simulink model "Full_Model_D_R6"  (R2013a)
settings: Solver=ode45  StartTime=0.0  StopTime=sim_length  MaxStep=1e-4  RelTol=1e-3
values from neighbouring files (symbols this model uses):
  A_Height_d = [1  0.02  0.00306066709295; 0  1  0.292172619905; 0  0  0.751477293075]    [Height_Controller_SS_D_Data.mat]    (also in Height_Controller_Sample_Time.m = A_d)
  A_Roll_d = [1  0.02  0.00957373027909; 0  1  0.913912481482; 0  0  0.751477293075]    [Roll_Controller_SS_D_Data.mat]    (also in Roll_Controller_Sample_Time.m = A_d)
  A_x_d = [1  0.725237004499; 0  0.506103765926]    [xy_Controller_PD_D_Data.mat]    (also in xy_Controller_PID_D_Data.mat; xy_Controller_Sample_Time.m = sys_d.a; xy_Controller_Sample_Time_2.m = sys_d.a)
  A_Yaw_d = [1  0.02  0.000714353321797; 0  1  0.0681924806681; 0  0  0.751477293075]    [Yaw_Controller_SS_D_Data.mat]    (also in Yaw_Controller_Sample_Time.m = A_d)
  B_Height_d = [0.000298297262238 0.0437238156136 0.248522706925]    [Height_Controller_SS_D_Data.mat]    (also in Height_Controller_Sample_Time.m = B_d)
  B_Roll_d = [0.000933070289885 0.136767575416 0.248522706925]    [Roll_Controller_SS_D_Data.mat]    (also in Roll_Controller_Sample_Time.m = B_d)
  B_x_d = [3.95796081795 7.11457501414]    [xy_Controller_PD_D_Data.mat]    (also in xy_Controller_PID_D_Data.mat; xy_Controller_Sample_Time.m = sys_d.b; xy_Controller_Sample_Time_2.m = sys_d.b)
  B_Yaw_d = [7.15569400366e-05 0.0103985455153 0.248522706925]    [Yaw_Controller_SS_D_Data.mat]    (also in Yaw_Controller_Sample_Time.m = B_d)
  C_Height_d = [1 0 0]    [Height_Controller_SS_D_Data.mat]    (also in Height_Controller_Sample_Time.m = C_d)
  C_Roll_d = [1  0  0; 0  1  0]    [Roll_Controller_SS_D_Data.mat]    (also in Roll_Controller_Sample_Time.m = C_d)
  C_x_d = [1 0]    [xy_Controller_PD_D_Data.mat]    (also in xy_Controller_PID_D_Data.mat; xy_Controller_Sample_Time.m = sys_d.c; xy_Controller_Sample_Time_2.m = sys_d.c)
  C_Yaw_d = [1  0  0; 0  1  0]    [Yaw_Controller_SS_D_Data.mat]    (also in Yaw_Controller_Sample_Time.m = C_d)
  coeff_speed1 = [-597.852411164 15567.4958959 -112629.522245 385376.825444 -722286.582234 762343.511164 -424427.181206 96698.0914793]    [Model_Parameters.mat]
  coeff_speed2 = [-33137.8630803 359389.817861 -1655728.0128 4197976.53355 -6322358.45977 5652250.74311 -2774846.33743 576528.840344]    [Model_Parameters.mat]
  coeff_speed3 = [-11936.4686056 137218.314774 -666283.661319 1770733.67902 -2780453.20018 2577948.57948 -1305141.01347 277978.291866]    [Model_Parameters.mat]
  coeff_speed4 = [-6669.45808334 79913.0612752 -401123.444791 1094619.31774 -1754742.75761 1652252.04897 -844945.337957 180729.993964]    [Model_Parameters.mat]
  coeff_thrust1 = [411.996230985 -4101.92524784 17203.3662669 -39329.1303747 52812.747408 -41528.8245566 17635.526271 -3103.13769268]    [Model_Parameters.mat]
  coeff_thrust2 = [3.52133616408 187.041584587 -1860.27738451 7135.94114535 -14212.0789042 15650.5208884 -9059.28758852 2154.75680942]    [Model_Parameters.mat]
  coeff_thrust3 = [-509.084474191 5539.72556164 -25664.1372161 65589.3028623 -99834.0669633 90481.3955019 -45198.9623282 9597.06354792]    [Model_Parameters.mat]
  coeff_thrust4 = [270.975135723 -2599.21496486 10453.4946669 -22770.946547 28872.4244579 -21147.1170047 8185.59308918 -1264.84197054]    [Model_Parameters.mat]
  Drag = 4.45306861536e-07    [Model_Parameters.mat]
  F_Roll_d = A_Roll_d-G_Roll_d*C_Roll_d    [Script_Controller_Sample_Time.m]    (also in Test_Controller_Sample_Time.m)
  F_yIntercept = -10.4432883127    [Model_Parameters.mat]
  Feed_Forward_Height_d = 2    [Height_Controller_SS_D_Data.mat]    (also in Height_Controller_Sample_Time.m)
  Feed_Forward_Roll_d = 0.125    [Roll_Controller_SS_D_Data.mat]    (also in Roll_Controller_Sample_Time.m)
  Feed_Forward_Yaw_d = 0    [Yaw_Controller_SS_D_Data.mat]    (also in Yaw_Controller_Sample_Time.m)
  g = 9.81    [Model_Parameters.mat]
  G_Height_d = [1.56504668046 34.0074022073 8.86962171802]    [Height_Controller_SS_D_Data.mat]    (also in Height_Controller_Sample_Time.m = place(A_d',C_d',P)')
  G_Roll_d = [0.251889913145  0.0200094814614; 0.229685260441  0.24715204306; -0.000711541775691  -9.30790483026e-05]    [Roll_Controller_SS_D_Data.mat]    (also in Roll_Controller_Sample_Time.m = place(A_d',C_d',P)')
  G_x_d = [-0.193896234074 0.15962315642]    [xy_Controller_PD_D_Data.mat]    (also in xy_Controller_PID_D_Data.mat; xy_Controller_Sample_Time.m = place(A_x_d',C_x_d',P)'; xy_Controller_Sample_Time_2.m = place(A_x_d',C_x_d',P)')
  G_Yaw_d = [0.242030648398  0.0200584166088; 0.0044560948779  0.235341919238; -0.000643549416335  -0.000818909263128]    [Yaw_Controller_SS_D_Data.mat]    (also in Yaw_Controller_Sample_Time.m = place(A_d',C_d',P)')
  I_Phi = 0.127422725814    [Model_Parameters.mat]
  I_Psi = 0.236966962973    [Model_Parameters.mat]
  I_Theta = 0.122104044652    [Model_Parameters.mat]
  J = 8e-08    [Model_Parameters.mat]
  K_Height_d = [2.7513802614 0.716922726377 0.637441613793]    [Height_Controller_SS_D_Data.mat]    (also in Height_Controller_Sample_Time.m = K_Height_Reg(1:end-1))
  K_Height_i = -2.03246593773    [Height_Controller_SS_D_Data.mat]    (also in Height_Controller_Sample_Time.m = K_Height_Reg(end))
  K_Roll_d = [2.67637429311 0.450684169535 1.07098831744]    [Roll_Controller_SS_D_Data.mat]    (also in Roll_Controller_Sample_Time.m = K_Roll_Reg(1:end-1))
  K_Roll_i = -2.24117965782    [Roll_Controller_SS_D_Data.mat]    (also in Roll_Controller_Sample_Time.m = K_Roll_Reg(end))
  K_Yaw_d = [1.55130112498 0.960619912039 0.23556072791]    [Yaw_Controller_SS_D_Data.mat]    (also in Yaw_Controller_Sample_Time.m = K_Yaw_Reg(1:end-1))
  K_Yaw_i = -1.12834490639    [Yaw_Controller_SS_D_Data.mat]    (also in Yaw_Controller_Sample_Time.m = K_Yaw_Reg(end))
  Kd_x = 0    [xy_Controller_PD_D_Data.mat]    (also in xy_Controller_PID_D_Data.mat = 0.0186150358972; xy_Controller_Sample_Time.m = get(C,'Kd'); xy_Controller_Sample_Time_2.m = get(C,'Kd'))
  Kd_y = 0    [xy_Controller_PD_D_Data.mat]    (also in xy_Controller_PID_D_Data.mat = 0.0186150358972; xy_Controller_Sample_Time.m = Kd_x; xy_Controller_Sample_Time_2.m = Kd_x)
  Kf = 9.48907430341    [Model_Parameters.mat]
  Ki_x = 0.000229999504243    [xy_Controller_PD_D_Data.mat]    (also in xy_Controller_PID_D_Data.mat = 0.000234605659833; xy_Controller_Sample_Time.m = get(C,'Ki'); xy_Controller_Sample_Time_2.m = get(C,'Ki'))
  Ki_y = 0.000229999504243    [xy_Controller_PD_D_Data.mat]    (also in xy_Controller_PID_D_Data.mat = 0.000234605659833; xy_Controller_Sample_Time.m = Ki_x; xy_Controller_Sample_Time_2.m = Ki_x)
  Kp_x = 0.032529495388    [xy_Controller_PD_D_Data.mat]    (also in xy_Controller_PID_D_Data.mat = 0.0333125747447; xy_Controller_Sample_Time.m = get(C,'Kp'); xy_Controller_Sample_Time_2.m = get(C,'Kp'))
  Kp_y = 0.032529495388    [xy_Controller_PD_D_Data.mat]    (also in xy_Controller_PID_D_Data.mat = 0.0333125747447; xy_Controller_Sample_Time.m = Kp_x; xy_Controller_Sample_Time_2.m = Kp_x)
  Kw = 501.513336009    [Model_Parameters.mat]
  L = 0.338    [Model_Parameters.mat]
  Mass = 2.26    [Model_Parameters.mat]
  Motor_TimeConstant = 0.07    [Model_Parameters.mat]
  NoiseDelay = 0    [All_Controller_Sample_Time.m]
  NoiseMean = 0    [All_Controller_Sample_Time.m]
  omega_0 = (0-F_yIntercept)/Kf    [Test_Controller_Sample_Time.m]    (also in Yaw_Controller_Sample_Time.m = 520)
  omega_Lim = (0-F_yIntercept)/Kf    [Test_Controller_Sample_Time.m]
  Phi_IC = (0/180)*pi    (= 0)    [Test_Controller_Sample_Time.m]
  Pitch_Setpoint = 0    [Test_Controller_Sample_Time.m]
  PropDelay = 0    [All_Controller_Sample_Time.m]
  Psi_IC = (0/180)*pi    (= 0)    [Test_Controller_Sample_Time.m]
  PWM_LimHigher = 2    [Test_Controller_Sample_Time.m]
  PWM_LimLower = 1.1    [Test_Controller_Sample_Time.m]
  Speed_yIntercept = -347.939581678    [Model_Parameters.mat]
  Tau_filter1 = 0.5    [All_Controller_Sample_Time.m]
  Theta_IC = (5/180)*pi    (= 0.0872664625997)    [Test_Controller_Sample_Time.m]
  Ts = 20e-3    (= 0.02)    [All_Controller_Sample_Time.m]
  Ts2 = 1    [All_Controller_Sample_Time.m]
  ViscousDamping = 36*sin(20/180*pi)/8    [All_Controller_Sample_Time.m]
  Yaw_Setpoint = 0    [Test_Controller_Sample_Time.m]
undefined symbols (not defined in the file or in its folder): DiscIntNeverNeededParam
libraries: simulink x9, commnoisgen2 x7
(part 2 of 2)

== system Full_Model_D_R6/Non Linear Quadcopter Model/Motor Model 4 ==
  Duty Cycle : Inport
  1/ Motor Time Constant : Gain  Gain=1/Motor_TimeConstant
  Fcn : Fcn  Expr=coeff_speed4(1)*u(1)^7 + coeff_speed4(2)*u(1)^6+coeff_speed4(3)*u(1)^5 + coeff_speed4(4)*u(1)^4+ coeff_speed4(5)*u(1)^3 +coeff_speed4(6)*u(1)^2+coeff_speed4(7)*u(1)+coeff_speed4(8)
  Fcn1 : Fcn  Expr=coeff_thrust4(1)*u(1)^7 + coeff_thrust4(2)*u(1)^6+coeff_thrust4(3)*u(1)^5 + coeff_thrust4(4)*u(1)^4+ coeff_thrust4(5)*u(1)^3 +coeff_thrust4(6)*u(1)^2+coeff_thrust4(7)*u(1)+coeff_thrust4(8)
  Manual Switch : ManualSwitch
  Manual Switch1 : ManualSwitch  CurrentSetting=0
  Motor 4 : Integrator  InitialCondition=omega_0  LimitOutput=on  LowerSaturationLimit=omega_Lim
  Motor Speed Slope : Gain  Gain=Kw
  Motor Speed Slope1 : Gain  Gain=Kw
  Motor Thrust Slope : Gain  Gain=Kf
  Sum2 : Sum  Inputs=++|
  Sum3 : Sum  Inputs=|+-
  Sum4 : Sum  Inputs=|++
  To Workspace10 : ToWorkspace  VariableName=MotorSpeed1  SampleTime=-1  SaveFormat=Timeseries
  y-Intercept of the  Motor Force Trendline : Constant  Value=F_yIntercept
  y-Intercept of the  Motor Speed Trendline : Constant  Value=Speed_yIntercept
  Thrust : Outport
  Acceleration : Outport  Port=2
  Speed : Outport  Port=3
  wires:
  Motor Thrust Slope/1 -> Sum2/2  "Thrust"
  Motor 4/1 -> Sum3/2, Fcn1/1, Fcn/1, Motor Speed Slope/1, Motor Thrust Slope/1
  Duty Cycle/1 -> Sum3/1
  Sum3/1 -> 1/ Motor Time Constant/1
  1/ Motor Time Constant/1 -> Motor 4/1, Motor Speed Slope1/1
  Motor Speed Slope/1 -> Sum4/1
  Motor Speed Slope1/1 -> Acceleration/1
  Sum2/1 -> Manual Switch1/2
  y-Intercept of the  Motor Force Trendline/1 -> Sum2/1
  Sum4/1 -> Manual Switch/2, To Workspace10/1
  y-Intercept of the  Motor Speed Trendline/1 -> Sum4/2
  Manual Switch/1 -> Speed/1
  Fcn/1 -> Manual Switch/1
  Manual Switch1/1 -> Thrust/1
  Fcn1/1 -> Manual Switch1/1

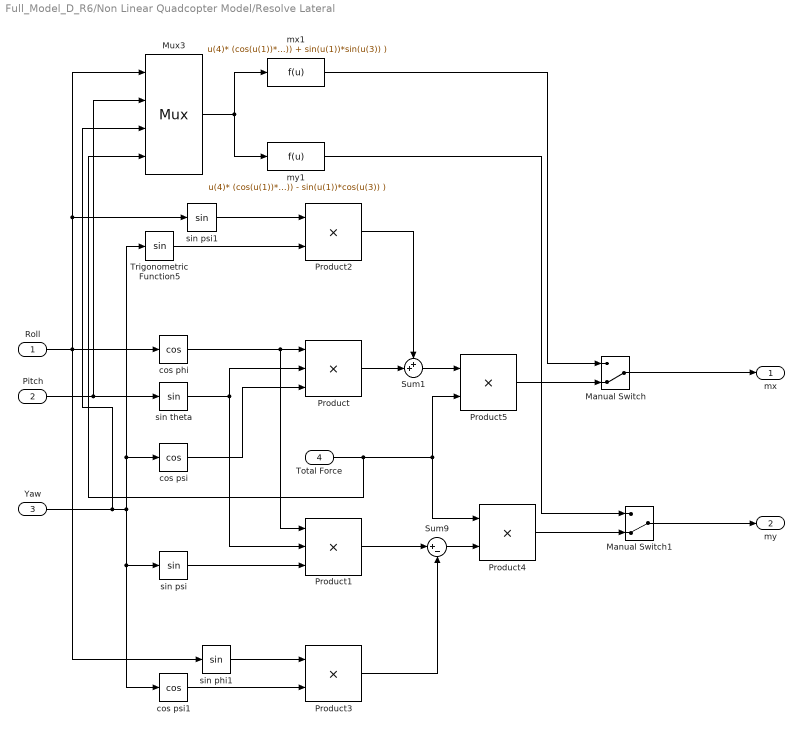
== system Full_Model_D_R6/Non Linear Quadcopter Model/Resolve Lateral ==
  Roll : Inport
  Pitch : Inport  Port=2
  Yaw : Inport  Port=3
  Total Force : Inport  Port=4
  Manual Switch : ManualSwitch  CurrentSetting=0
  Manual Switch1 : ManualSwitch  CurrentSetting=0
  Mux3 : Mux
      settings: DisplayOption=signals
  Product : Product  Inputs=3
  Product1 : Product  Inputs=3
  Product{2..5} (4 alike) : Product
  Sum1 : Sum  Inputs=++|
  Sum9 : Sum  Inputs=|+-
  Trigonometric Function5 : Trigonometry
  cos phi : Trigonometry  Operator=cos
  cos psi : Trigonometry  Operator=cos
  cos psi1 : Trigonometry  Operator=cos
  mx1 : Fcn  Expr=u(4)* (cos(u(1))*sin(u(2))*cos(u(3)) + sin(u(1))*sin(u(3)) )
  my1 : Fcn  Expr=u(4)* (cos(u(1))*sin(u(2))*sin(u(3)) - sin(u(1))*cos(u(3)) )
  sin phi1 : Trigonometry
  sin psi : Trigonometry
  sin psi1 : Trigonometry
  sin theta : Trigonometry
  mx : Outport
  my : Outport  Port=2
  wires:
  Product/1 -> Sum1/2
  Product1/1 -> Sum9/1
  cos phi/1 -> Product1/1, Product/1
  Pitch/1 -> Mux3/2, sin theta/1
  sin theta/1 -> Product/2, Product1/2
  cos psi/1 -> Product/3
  sin psi/1 -> Product1/3
  Sum1/1 -> Product5/1
  Product5/1 -> Manual Switch/2
  Product2/1 -> Sum1/1
  Total Force/1 -> Mux3/4, Product5/2, Product4/1
  Product4/1 -> Manual Switch1/2
  Sum9/1 -> Product4/2
  Product3/1 -> Sum9/2
  Trigonometric Function5/1 -> Product2/2
  cos psi1/1 -> Product3/2
  Yaw/1 -> Mux3/3, sin psi/1, cos psi1/1, cos psi/1, Trigonometric Function5/1
  sin psi1/1 -> Product2/1
  Roll/1 -> cos phi/1, Mux3/1, sin psi1/1, sin phi1/1
  sin phi1/1 -> Product3/1
  Mux3/1 -> my1/1, mx1/1
  mx1/1 -> Manual Switch/1
  my1/1 -> Manual Switch1/1
  Manual Switch/1 -> mx/1
  Manual Switch1/1 -> my/1

== system Full_Model_D_R6/Non Linear Quadcopter Model/Resolve Vertical ==
  Total Force : Inport
  Total Force1 : Inport  Port=2
  Roll : Inport  Port=3
  Product : Product  Inputs=3
  Trigonometric Function : Trigonometry  Operator=cos
  Trigonometric Function1 : Trigonometry  Operator=cos
  Vertical Force : Outport
  wires:
  Trigonometric Function/1 -> Product/1
  Total Force/1 -> Product/3
  Roll/1 -> Trigonometric Function1/1
  Total Force1/1 -> Trigonometric Function/1
  Product/1 -> Vertical Force/1
  Trigonometric Function1/1 -> Product/2

== system Full_Model_D_R6/Pitch Controller and Observer/Difference Equations ==
  Setpoint : Inport
  xhat1 : Inport  Port=2
  xhat2 : Inport  Port=3
  xhat3 : Inport  Port=4
  Delay1 : Delay  DelayLength=1
  Mux : Mux  Inputs=5
  Mux3 : Mux  Inputs=3
  Roll Integator : Fcn  Expr=u(1) + ( -K_Roll_i*Ts*( u(2)-u(3) ))  SampleTime=Ts
  Roll Regulator : Fcn  Expr=Feed_Forward_Roll_d*u(1)+u(2)-K_Roll_d(1)*u(3)-K_Roll_d(2)*u(4)-K_Roll_d(3)*u(5)  SampleTime=Ts
  u1 : Outport
  wires:
  Delay1/1 -> Mux3/1
  Mux/1 -> Roll Regulator/1
  xhat2/1 -> Mux/4
  xhat3/1 -> Mux/5
  xhat1/1 -> Mux/3, Mux3/3
  Setpoint/1 -> Mux3/2, Mux/1
  Roll Regulator/1 -> u1/1
  Roll Integator/1 -> Delay1/1, Mux/2  "v(k)"
  Mux3/1 -> Roll Integator/1

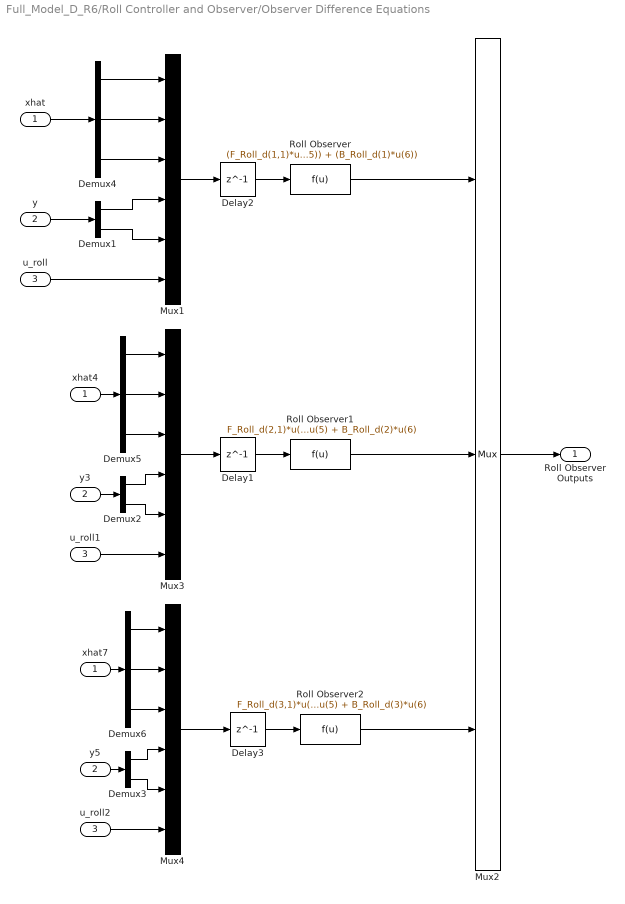
== system Full_Model_D_R6/Roll Controller and Observer/Observer Difference Equations ==
  xhat : Inport
  y : Inport  Port=2
  u_roll : Inport  Port=3
  Delay1 : Delay  DelayLength=1
  Delay2 : Delay  DelayLength=1
  Delay3 : Delay  DelayLength=1
  Demux1 : Demux  Outputs=2
  Demux2 : Demux  Outputs=2
  Demux3 : Demux  Outputs=2
  Demux4 : Demux  Outputs=3
  Demux5 : Demux  Outputs=3
  Demux6 : Demux  Outputs=3
  Mux1 : Mux  Inputs=6
  Mux2 : Mux  Inputs=3
  Mux3 : Mux  Inputs=6
  Mux4 : Mux  Inputs=6
  Roll Observer : Fcn  Expr=(F_Roll_d(1,1)*u(1) ) + (F_Roll_d(1,2)*u(2)) + (F_Roll_d(1,3)*u(3)) + (G_Roll_d(1,1)*u(4)) + (G_Roll_d(1,2)*u(5)) + (B_Roll_d(1)*u(6))  SampleTime=Ts
  Roll Observer1 : Fcn  Expr=F_Roll_d(2,1)*u(1) + F_Roll_d(2,2)*u(2) + F_Roll_d(2,3)*u(3) + G_Roll_d(2,1)*u(4) + G_Roll_d(2,2)*u(5) + B_Roll_d(2)*u(6)  SampleTime=Ts
  Roll Observer2 : Fcn  Expr=F_Roll_d(3,1)*u(1) + F_Roll_d(3,2)*u(2) + F_Roll_d(3,3)*u(3) + G_Roll_d(3,1)*u(4) + G_Roll_d(3,2)*u(5) + B_Roll_d(3)*u(6)  SampleTime=Ts
  u_roll1 : InportShadow  Port=3
  u_roll2 : InportShadow  Port=3
  xhat4 : InportShadow
  xhat7 : InportShadow
  y3 : InportShadow  Port=2
  y5 : InportShadow  Port=2
  Roll Observer Outputs : Outport
  wires:
  u_roll/1 -> Mux1/6
  y/1 -> Demux1/1
  Roll Observer/1 -> Mux2/1
  Mux1/1 -> Delay2/1
  Delay2/1 -> Roll Observer/1
  Mux2/1 -> Roll Observer Outputs/1
  Mux3/1 -> Delay1/1
  Delay1/1 -> Roll Observer1/1
  y3/1 -> Demux2/1
  u_roll1/1 -> Mux3/6
  y5/1 -> Demux3/1
  u_roll2/1 -> Mux4/6
  Delay3/1 -> Roll Observer2/1
  Mux4/1 -> Delay3/1
  Roll Observer2/1 -> Mux2/3
  Roll Observer1/1 -> Mux2/2
  Demux1/1 -> Mux1/4
  Demux1/2 -> Mux1/5
  Demux2/1 -> Mux3/4
  Demux2/2 -> Mux3/5
  Demux3/1 -> Mux4/4
  Demux3/2 -> Mux4/5
  xhat/1 -> Demux4/1
  Demux4/1 -> Mux1/1
  Demux4/3 -> Mux1/3
  Demux4/2 -> Mux1/2
  xhat4/1 -> Demux5/1
  Demux5/2 -> Mux3/2
  Demux5/1 -> Mux3/1
  Demux5/3 -> Mux3/3
  xhat7/1 -> Demux6/1
  Demux6/2 -> Mux4/2
  Demux6/3 -> Mux4/3
  Demux6/1 -> Mux4/1

== system Full_Model_D_R6/Roll Controller and Observer/Regulator Difference Equations ==
  Setpoint : Inport
  Observed Inputs : Inport  Port=2
  Delay1 : Delay  DelayLength=1
  Demux2 : Demux  Outputs=3
  Mux : Mux  Inputs=5
  Mux3 : Mux  Inputs=3
  Roll Integator : Fcn  Expr=u(1) + ( -K_Roll_i*Ts*( u(2)-u(3) ))  SampleTime=Ts
  Roll Regulator : Fcn  Expr=Feed_Forward_Roll_d*u(1)+u(2)-K_Roll_d(1)*u(3)-K_Roll_d(2)*u(4)-K_Roll_d(3)*u(5)  SampleTime=Ts
  u1 : Outport
  wires:
  Delay1/1 -> Mux3/1
  Mux/1 -> Roll Regulator/1
  Setpoint/1 -> Mux3/2, Mux/1  "r(k)"
  Roll Regulator/1 -> u1/1
  Roll Integator/1 -> Delay1/1, Mux/2  "v(k)"
  Mux3/1 -> Roll Integator/1
  Demux2/1 -> Mux3/3, Mux/3  "x1hat"
  Demux2/2 -> Mux/4  "x2hat"
  Demux2/3 -> Mux/5  "x3hat"
  Observed Inputs/1 -> Demux2/1

== system Full_Model_D_R6/Subsystem/Pitch Sensor Filter ==
  Pitch Angle : Inport
  Pitch Rate : Inport  Port=2
  Delay1 : Delay  DelayLength=1  SampleTime=Ts
  Delay2 : Delay  DelayLength=1  SampleTime=Ts
  Delay3 : Delay  DelayLength=1  SampleTime=Ts
  Filter Gain : Gain  Gain=1 /(Ts+2*Tau_filter1)  SampleTime=Ts
  Mux3 : Mux  Inputs=5
  Roll Filter : Fcn  Expr=Ts*( u(1) + u(2) + Tau_filter1*(u(3) +u(4) ) ) - (Ts-2*Tau_filter1)*(u(5))  SampleTime=Ts
  Sampler : Gain  SampleTime=Ts
  Sampler1 : Gain  SampleTime=Ts
  Pitch Filtered : Outport
  wires:
  Pitch Rate/1 -> Sampler/1
  Mux3/1 -> Filter Gain/1
  Delay1/1 -> Mux3/2
  Delay2/1 -> Mux3/4
  Sampler/1 -> Delay2/1, Mux3/3
  Pitch Angle/1 -> Sampler1/1
  Sampler1/1 -> Delay1/1, Mux3/1
  Roll Filter/1 -> Pitch Filtered/1, Delay3/1  "v(k)"
  Filter Gain/1 -> Roll Filter/1
  Delay3/1 -> Mux3/5

== system Full_Model_D_R6/Subsystem/Roll Sensor Filter1 ==
  Roll Angle : Inport
  Roll Rate : Inport  Port=2
  Delay1 : Delay  DelayLength=1  SampleTime=Ts
  Delay2 : Delay  DelayLength=1  SampleTime=Ts
  Delay3 : Delay  DelayLength=1  SampleTime=Ts
  Filter Gain : Gain  Gain=1 /(Ts+2*Tau_filter1)  SampleTime=Ts
  Mux3 : Mux  Inputs=5
  Roll Filter : Fcn  Expr=Ts*( u(1) + u(2) + Tau_filter1*(u(3) +u(4) ) ) - (Ts-2*Tau_filter1)*(u(5))  SampleTime=Ts
  Sampler : Gain  SampleTime=Ts
  Sampler1 : Gain  SampleTime=Ts
  Roll Filtered : Outport
  wires:
  Roll Rate/1 -> Sampler/1
  Mux3/1 -> Filter Gain/1
  Delay1/1 -> Mux3/2
  Delay2/1 -> Mux3/4
  Sampler/1 -> Delay2/1, Mux3/3
  Roll Angle/1 -> Sampler1/1
  Sampler1/1 -> Delay1/1, Mux3/1
  Roll Filter/1 -> Roll Filtered/1, Delay3/1  "v(k)"
  Filter Gain/1 -> Roll Filter/1
  Delay3/1 -> Mux3/5

== system Full_Model_D_R6/Yaw Controller and Observer/Difference Equations ==
  Setpoint : Inport
  xhat1 : Inport  Port=2
  xhat2 : Inport  Port=3
  xhat3 : Inport  Port=4
  Delay1 : Delay  DelayLength=1
  Mux : Mux  Inputs=5
  Mux3 : Mux  Inputs=3
  Roll Integator : Fcn  Expr=u(1) + ( -K_Yaw_i*Ts*( u(2)-u(3) ))  SampleTime=Ts
  Roll Regulator : Fcn  Expr=Feed_Forward_Yaw_d*u(1)+u(2)-K_Yaw_d(1)*u(3)-K_Yaw_d(2)*u(4)-K_Yaw_d(3)*u(5)  SampleTime=Ts
  u1 : Outport
  wires:
  Delay1/1 -> Mux3/1
  Mux/1 -> Roll Regulator/1
  xhat2/1 -> Mux/4
  xhat3/1 -> Mux/5
  xhat1/1 -> Mux/3, Mux3/3
  Setpoint/1 -> Mux3/2, Mux/1
  Roll Regulator/1 -> u1/1
  Roll Integator/1 -> Delay1/1, Mux/2  "v(k)"
  Mux3/1 -> Roll Integator/1
